simulink model "H"  (R2013a)
settings: Solver=FixedStepDiscrete  StartTime=0.0  StopTime=10.0  RelTol=1e-3
settings Model: Creator=Élio  LastModifiedBy=Élio

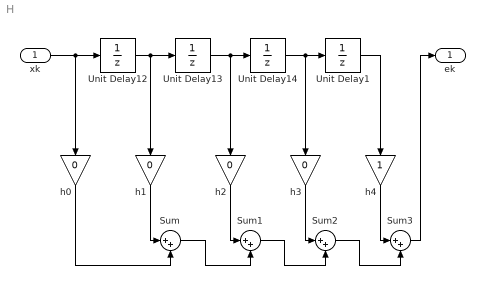
== system H ==
  xk : Inport
  Sum{,1..3} (4 alike) : Sum  Inputs=|++
  Unit Delay{1,12..14} (4 alike) : UnitDelay  SampleTime=-1
  h{0..3} (4 alike) : Gain  Gain=0
  h4 : Gain
  ek : Outport
  wires:
  Unit Delay12/1 -> Unit Delay13/1, h1/1
  Unit Delay13/1 -> Unit Delay14/1, h2/1
  Unit Delay14/1 -> Unit Delay1/1, h3/1
  h1/1 -> Sum/1
  h0/1 -> Sum/2
  xk/1 -> Unit Delay12/1, h0/1
  Sum/1 -> Sum1/2
  h2/1 -> Sum1/1
  h3/1 -> Sum2/1
  Sum1/1 -> Sum2/2
  Unit Delay1/1 -> h4/1
  h4/1 -> Sum3/1
  Sum2/1 -> Sum3/2
  Sum3/1 -> ek/1
